simulink model "FOSWEC2"  (R2025b)
settings: Solver=FixedStepAuto  StartTime=0.0  StopTime=Inf  FixedStep=Ts  RelTol=1e-3
values from neighbouring files (symbols this model uses):
  ExcelGains = table2array(ExcelGains)    [initFOSWEC2.m]
  gainTstep = 1.55*20    (= 31)    [initFOSWEC2.m]
  stepTime = 10    [initFOSWEC2.m]
  T = 5    [initFOSWEC2.m]
  Ts = 0.001    [initFOSWEC2.m]
undefined symbols (not defined in the file or in its folder): aft, aftBus_V, aftCurrent_A, aftFlap_deg, aftFlap_Nm, aftPos_rad, aftPower_W, aftRotVel_radpers, aftRotVelFilt_radpers, aftRotVelfromPos_radpers, aftTarget_A, aftTarget_Nm, aftTorque_Nm, bow, bowBus_V, bowCurrent_A, bowFlap_deg, bowFlap_Nm, bowPos_rad, bowPower_W, bowRotVel_radpers, bowRotVelFilt_radpers, bowRotVelfromPos_radpers, bowTarget_A, bowTarget_Nm, bowTorque_Nm, rampTime
libraries: slrealtimeethercatlib x30, simulink x20, slrealtimeloglib x10, dspfdesign x4, cstblocks x2, slrealtimeptplib x1, dspsrcs4 x1
settings Model: Creator=HWRL user  LastModifiedBy=bosmab
settings SolverCC: ConcurrentTasks=on  PositivePriorityOrder=on
settings DataIOCC: ExternalInput=ds  LoadExternalInput=on
settings OptimizationCC: BlockReduction=off  OptimizeBlockIOStorage=off  ReuseModelBlockBuffer=off
settings DebuggingCC: TasksWithSamePriorityMsg=none  ParameterPrecisionLossMsg=none
settings HardwareCC: ProdBitPerLong=64.0  ProdLongLongMode=on  ProdHWDeviceType=Intel->x86-64 (Linux 64)
settings RTWCC: SystemTargetFile=speedgoat.tlc  TemplateMakefile=slrealtime_default_tmf  RTWVerbose=off  Toolchain=Simulink Real-Time Toolchain  BuildConfiguration=Faster Runs  CodeExecutionProfiling=on  TargetLang=C++  GPUComputeCapability=3.5  Description=Speedgoat Real-Time Target Machine
settings SimulinkRealTimeTargetCC: SLRTFileLogMaxRuns=1.0  ExtModeMaxTrigDuration=10.0  ExtModeStaticAllocSize=1000000.0  ExtModeTransport=0.0  MultiwordLength=2048.0  DynamicStringBufferSize=256.0  PreserveMATLABNamespacesInGeneratedCode=on  SubcomponentCodeInterfacePackaging=Reusable function  InstructionSetFMA=off  LogToMDFFile=off

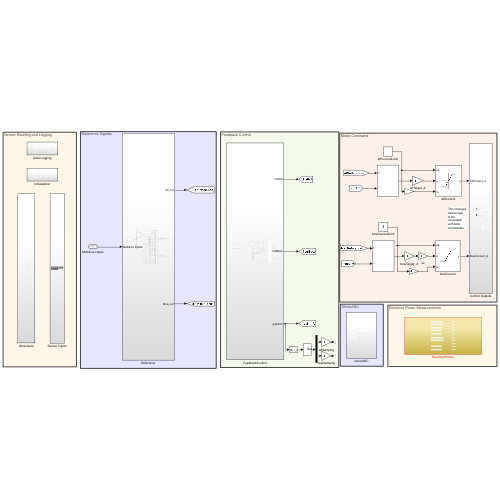
[thumbnail: Simulink's stored preview of the top-level diagram]
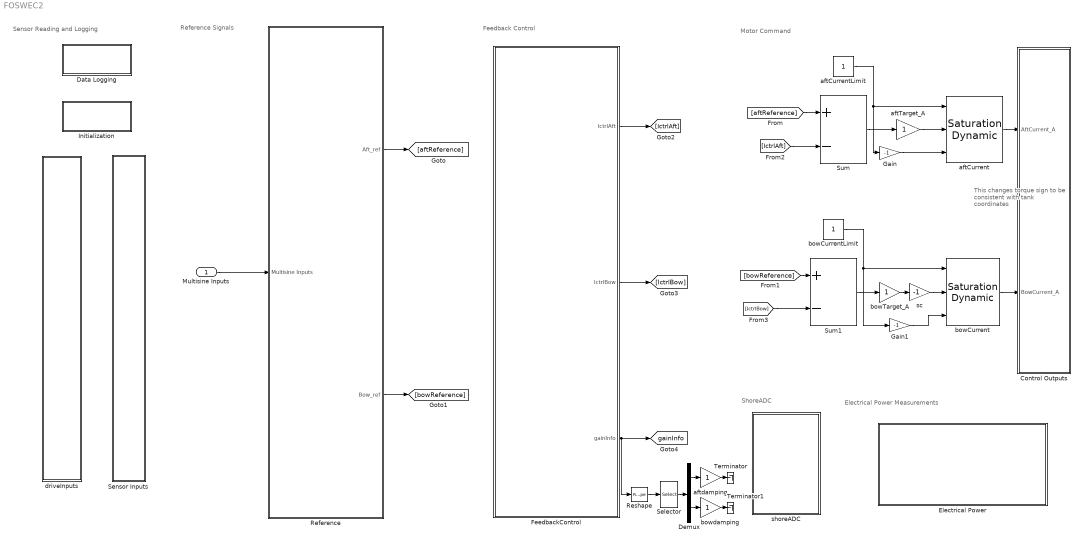
== system FOSWEC2 ==
  note: Electrical Power Measurements
  note: ShoreADC
  note: Sensor Reading and Logging
  note: Motor Command
  note: Feedback Control
  note: Reference Signals
  note: This changes torque sign to be consistent with tank coordinates
  Multisine Inputs : Inport  OutDataTypeStr=Bus: refSigs
  Control Outputs : Subsystem
  Data Logging : Subsystem
  Demux : Demux  Outputs=2
  Electrical Power : Subsystem
  FeedbackControl : Subsystem
  Gain : Gain  Gain=-1
  Gain1 : Gain  Gain=-1
  Initialization : Subsystem
  Reference : Subsystem
  Reshape : Reshape
  Selector : Selector  InputPortWidth=8  IndexOptions=Index vector (dialog)  Indices=[2 8]  OutputSizes=1
  Sensor Inputs : Subsystem
  Sum : Sum  Inputs=+-
  Sum1 : Sum  Inputs=+-
  Terminator : Terminator
  Terminator1 : Terminator
  aftCurrent : simulink/Discontinuities/Saturation Dynamic  OutMin=[]  OutMax=[]  OutDataTypeStr=Inherit: Same as second input  OutDataType=fixdt(1, 16)  OutScaling=2^-10  DoSatur=off
  aftCurrentLimit : Constant
  aftTarget_A : Gain
  aftdamping : Gain
  bowCurrent : simulink/Discontinuities/Saturation Dynamic  OutMin=[]  OutMax=[]  OutDataTypeStr=Inherit: Same as second input  OutDataType=fixdt(1, 16)  OutScaling=2^-10  DoSatur=off
  bowCurrentLimit : Constant
  bowTarget_A : Gain
  bowdamping : Gain
  driveInputs : Subsystem
  sc : Gain  Gain=-1
  shoreADC : Subsystem
  tag scope: gainInfo=global
  wires:
  Sum/1 -> aftTarget_A/1
  Gain/1 -> aftCurrent/3
  aftCurrentLimit/1 -> Gain/1, aftCurrent/1
  [IctrlBow] -> Sum1/2
  bowCurrentLimit/1 -> Gain1/1, bowCurrent/1
  Gain1/1 -> bowCurrent/3
  Sum1/1 -> bowTarget_A/1
  [aftReference] -> Sum/1
  FeedbackControl/1(IctrlAft) -> [IctrlAft]
  [IctrlAft] -> Sum/2
  FeedbackControl/2(IctrlBow) -> [IctrlBow]
  FeedbackControl/3(gainInfo) -> Reshape/1, [gainInfo]
  [bowReference] -> Sum1/1
  bowTarget_A/1 -> sc/1
  aftCurrent/1 -> Control Outputs/1(AftCurrent_A)
  bowCurrent/1 -> Control Outputs/2(BowCurrent_A)
  sc/1 -> bowCurrent/2
  aftTarget_A/1 -> aftCurrent/2
  Demux/1 -> aftdamping/1
  Demux/2 -> bowdamping/1
  aftdamping/1 -> Terminator/1
  bowdamping/1 -> Terminator1/1
  Reshape/1 -> Selector/1
  Selector/1 -> Demux/1
  Multisine Inputs/1 -> Reference/1(Multisine Inputs)
  Reference/1(Aft_ref) -> [aftReference]
  Reference/2(Bow_ref) -> [bowReference]

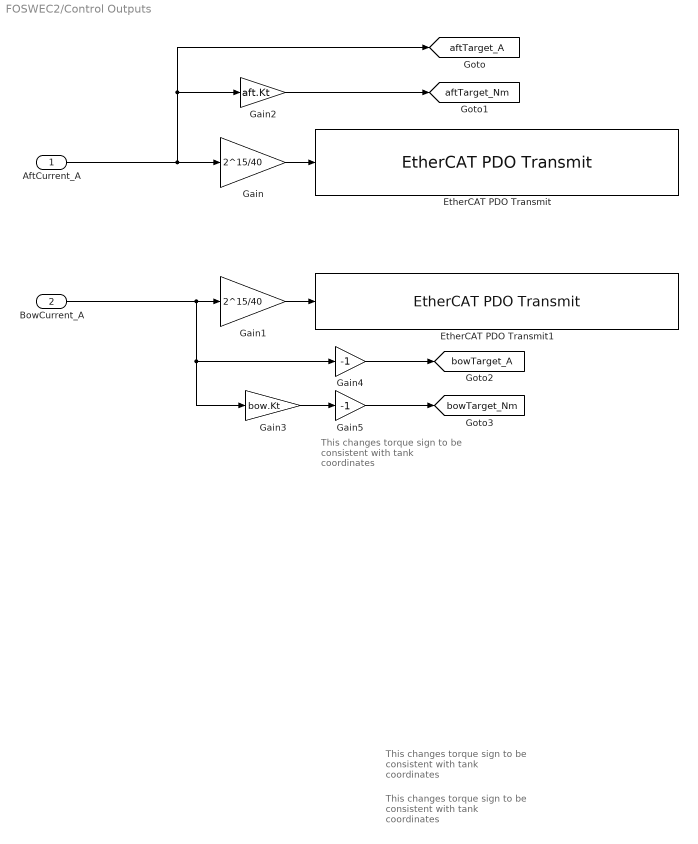
== system FOSWEC2/Control Outputs ==
  note: This changes torque sign to be consistent with tank coordinates
  note: This changes torque sign to be consistent with tank coordinates
  note: This changes torque sign to be consistent with tank coordinates
  AftCurrent_A : Inport
  BowCurrent_A : Inport  Port=2
  EtherCAT PDO Transmit : slrealtimeethercatlib/EtherCAT PDO Transmit  Priority=3  sig_name=Drive 8 (AMC).Module 1 (Default).PDO data to Slave.Target Current  sig_offset=792  sig_type=int16  type_size=16  sig_dim=1  device_id=0  sample_time=0.001000
  EtherCAT PDO Transmit1 : slrealtimeethercatlib/EtherCAT PDO Transmit  Priority=3  sig_name=Drive 4 (AMC).Module 1 (Default).PDO data to Slave.Target Current  sig_offset=648  sig_type=int16  type_size=16  sig_dim=1  device_id=0  sample_time=0.001000
  Gain : Gain  Gain=2^15/40  OutDataTypeStr=int16
  Gain1 : Gain  Gain=2^15/40  OutDataTypeStr=int16
  Gain2 : Gain  Gain=aft.Kt
  Gain3 : Gain  Gain=bow.Kt
  Gain4 : Gain  Gain=-1
  Gain5 : Gain  Gain=-1
  tag scope: aftTarget_A=global, aftTarget_Nm=global, bowTarget_A=global, bowTarget_Nm=global
  wires:
  Gain/1 -> EtherCAT PDO Transmit/1
  Gain1/1 -> EtherCAT PDO Transmit1/1
  Gain2/1 -> [aftTarget_Nm]
  Gain3/1 -> Gain5/1
  BowCurrent_A/1 -> Gain3/1, Gain4/1, Gain1/1
  AftCurrent_A/1 -> Gain/1, [aftTarget_A], Gain2/1
  Gain4/1 -> [bowTarget_A]
  Gain5/1 -> [bowTarget_Nm]

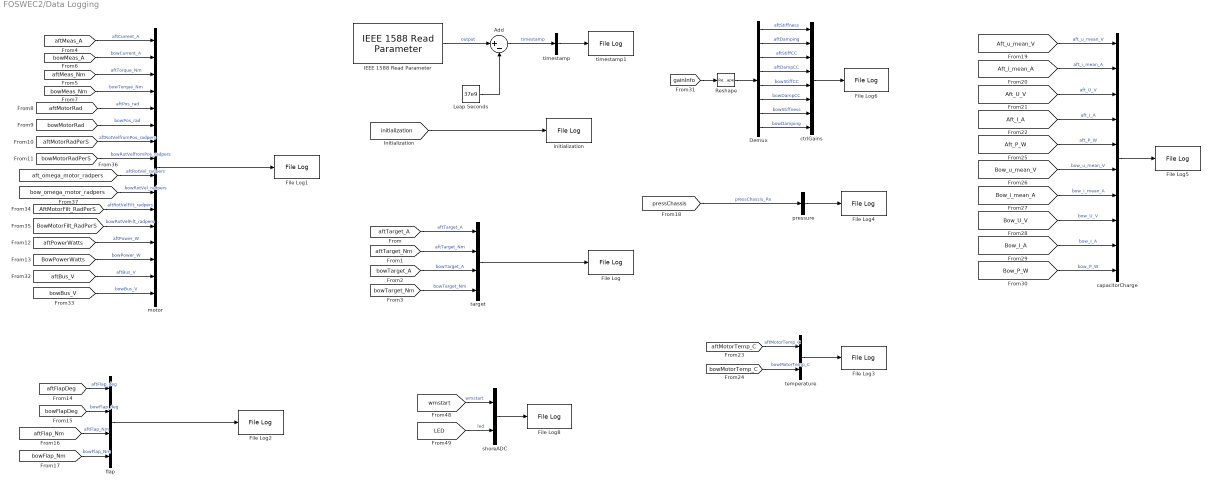
== system FOSWEC2/Data Logging ==
  Add : Sum  Inputs=|+-
  Demux : Demux  Outputs=8
  File Log{,1..6,8} (8 alike) : slrealtimeloglib/File Log  decimation=1  inputProcessing=Elements as channels (sample based)
  IEEE 1588 Read Parameter : slrealtimeptplib/IEEE 1588 Read Parameter  Priority=1  ID=1  param=1. System time (nanosecond)  sample_time=Ts
  Leap Seconds : Constant  Value=37e9
  Reshape : Reshape
  capacitorCharge : BusCreator  Inputs=10
  ctrlGains : BusCreator  Inputs=8
  flap : BusCreator  Inputs=aftFlap_deg,bowFlap_deg,aftFlap_Nm,bowFlap_Nm
  initialization : slrealtimeloglib/File Log  decimation=1  inputProcessing=Elements as channels (sample based)
  motor : BusCreator  Inputs=aftCurrent_A,bowCurrent_A,aftTorque_Nm,bowTorque_Nm,aftPos_rad,bowPos_rad,aftRotVelfromPos_radpers,bowRotVelfromPos_radpers,aftRotVel_radpers,bowRotVel_radpers,aftRotVelFilt_radpers,bowRotVelFilt_radpers,aftPower_W,bowPower_W,aftBus_V,bowBus_V
  pressure : BusCreator  Inputs=1
  shoreADC : BusCreator  Inputs=2
  target : BusCreator  Inputs=aftTarget_A,aftTarget_Nm,bowTarget_A,bowTarget_Nm
  temperature : BusCreator  Inputs=2
  timestamp : BusCreator  Inputs=timestamp
  timestamp1 : slrealtimeloglib/File Log  decimation=1  inputProcessing=Elements as channels (sample based)
  wires:
  Leap Seconds/1 -> Add/2
  IEEE 1588 Read Parameter/1 -> Add/1  "output"
  Add/1 -> timestamp/1  "timestamp"
  timestamp/1 -> timestamp1/1
  [initialization] -> initialization/1
  [aftTarget_A] -> target/1  "aftTarget_A"
  [aftTarget_Nm] -> target/2  "aftTarget_Nm"
  [bowTarget_A] -> target/3  "bowTarget_A"
  [bowTarget_Nm] -> target/4  "bowTarget_Nm"
  target/1 -> File Log/1
  [aftMeas_A] -> motor/1  "aftCurrent_A"
  [aftMeas_Nm] -> motor/3  "aftTorque_Nm"
  [bowMeas_A] -> motor/2  "bowCurrent_A"
  [bowMeas_Nm] -> motor/4  "bowTorque_Nm"
  [aftMotorRad] -> motor/5  "aftPos_rad"
  [bowMotorRad] -> motor/6  "bowPos_rad"
  motor/1 -> File Log1/1
  [aftMotorRadPerS] -> motor/7  "aftRotVelfromPos_radpers"
  [bowMotorRadPerS] -> motor/8  "bowRotVelfromPos_radpers"
  [aftPowerWatts] -> motor/13  "aftPower_W"
  [BowPowerWatts] -> motor/14  "bowPower_W"
  [aftMotorTemp_C] -> temperature/1  "aftMotorTemp_C"
  [bowMotorTemp_C] -> temperature/2  "bowMotorTemp_C"
  temperature/1 -> File Log3/1
  [gainInfo] -> Reshape/1
  Reshape/1 -> Demux/1
  Demux/1 -> ctrlGains/1  "aftStiffness"
  Demux/2 -> ctrlGains/2  "aftDamping"
  Demux/3 -> ctrlGains/3  "aftStiffCC"
  Demux/4 -> ctrlGains/4  "aftDampCC"
  Demux/5 -> ctrlGains/5  "bowStiffCC"
  Demux/6 -> ctrlGains/6  "bowDampCC"
  Demux/7 -> ctrlGains/7  "bowStiffness"
  Demux/8 -> ctrlGains/8  "bowDamping"
  ctrlGains/1 -> File Log6/1
  [aftBus_V] -> motor/15  "aftBus_V"
  [bowBus_V] -> motor/16  "bowBus_V"
  [AftMotorFilt_RadPerS] -> motor/11  "aftRotVelFilt_radpers"
  [BowMotorFilt_RadPerS] -> motor/12  "bowRotVelFilt_radpers"
  [bow_omega_motor_radpers] -> motor/10  "bowRotVel_radpers"
  [aft_omega_motor_radpers] -> motor/9  "aftRotVel_radpers"
  [wmstart] -> shoreADC/1  "wmstart"
  [LED] -> shoreADC/2  "led"
  shoreADC/1 -> File Log8/1
  [aftFlapDeg] -> flap/1  "aftFlap_deg"
  [bowFlapDeg] -> flap/2  "bowFlap_deg"
  flap/1 -> File Log2/1
  [aftFlap_Nm] -> flap/3  "aftFlap_Nm"
  [bowFlap_Nm] -> flap/4  "bowFlap_Nm"
  [pressChassis] -> pressure/1  "pressChassis_Pa"
  pressure/1 -> File Log4/1
  [Aft_u_mean_V] -> capacitorCharge/1  "aft_u_mean_V"
  [Aft_i_mean_A] -> capacitorCharge/2  "aft_i_mean_A"
  [Aft_U_V] -> capacitorCharge/3  "aft_U_V"
  [Aft_I_A] -> capacitorCharge/4  "aft_I_A"
  [Aft_P_W] -> capacitorCharge/5  "aft_P_W"
  [Bow_u_mean_V] -> capacitorCharge/6  "bow_u_mean_V"
  [Bow_i_mean_A] -> capacitorCharge/7  "bow_i_mean_A"
  [Bow_U_V] -> capacitorCharge/8  "bow_U_V"
  [Bow_I_A] -> capacitorCharge/9  "bow_I_A"
  [Bow_P_W] -> capacitorCharge/10  "bow_P_W"
  capacitorCharge/1 -> File Log5/1

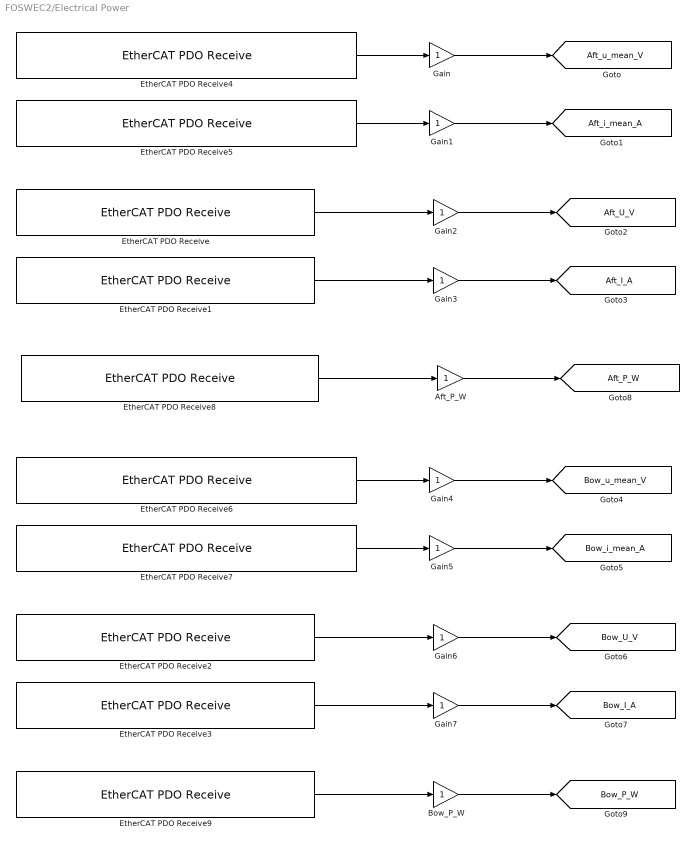
== system FOSWEC2/Electrical Power ==
  Aft_P_W : Gain  OutDataTypeStr=double
  Bow_P_W : Gain  OutDataTypeStr=double
  EtherCAT PDO Receive : slrealtimeethercatlib/EtherCAT PDO Receive  Priority=2  sig_name=Box 1 (GEN Series DAQ System).AftFlap.out.U.AftFlap.out.U_V  sig_offset=2096  sig_type=single  type_size=32  sig_dim=1  device_id=0  sample_time=0.001000
  EtherCAT PDO Receive1 : slrealtimeethercatlib/EtherCAT PDO Receive  Priority=2  sig_name=Box 1 (GEN Series DAQ System).AftFlap.out.I.AftFlap.out.I_V  sig_offset=2056  sig_type=single  type_size=32  sig_dim=1  device_id=0  sample_time=0.001000
  EtherCAT PDO Receive2 : slrealtimeethercatlib/EtherCAT PDO Receive  Priority=2  sig_name=Box 1 (GEN Series DAQ System).BowFlap.out.U.BowFlap.out.U_V  sig_offset=1776  sig_type=single  type_size=32  sig_dim=1  device_id=0  sample_time=0.001
  EtherCAT PDO Receive3 : slrealtimeethercatlib/EtherCAT PDO Receive  Priority=2  sig_name=Box 1 (GEN Series DAQ System).BowFlap.out.I.BowFlap.out.I_V  sig_offset=1736  sig_type=single  type_size=32  sig_dim=1  device_id=0  sample_time=0.001
  EtherCAT PDO Receive4 : slrealtimeethercatlib/EtherCAT PDO Receive  Priority=2  sig_name=Box 1 (GEN Series DAQ System).AftFlap.out.u_mean.AftFlap.out.u_mean_V  sig_offset=2176  sig_type=single  type_size=32  sig_dim=1  device_id=0  sample_time=0.001000
  EtherCAT PDO Receive5 : slrealtimeethercatlib/EtherCAT PDO Receive  Priority=2  sig_name=Box 1 (GEN Series DAQ System).AftFlap.out.i_mean.AftFlap.out.i_mean_V  sig_offset=2136  sig_type=single  type_size=32  sig_dim=1  device_id=0  sample_time=0.001000
  EtherCAT PDO Receive6 : slrealtimeethercatlib/EtherCAT PDO Receive  Priority=2  sig_name=Box 1 (GEN Series DAQ System).BowFlap.out.u_mean.BowFlap.out.u_mean_V  sig_offset=1856  sig_type=single  type_size=32  sig_dim=1  device_id=0  sample_time=0.001
  EtherCAT PDO Receive7 : slrealtimeethercatlib/EtherCAT PDO Receive  Priority=2  sig_name=Box 1 (GEN Series DAQ System).BowFlap.out.i_mean.BowFlap.out.i_mean_V  sig_offset=1816  sig_type=single  type_size=32  sig_dim=1  device_id=0  sample_time=0.001
  EtherCAT PDO Receive8 : slrealtimeethercatlib/EtherCAT PDO Receive  Priority=2  sig_name=Box 1 (GEN Series DAQ System).AftFlap.out.P.AftFlap.out.P_V  sig_offset=2216  sig_type=single  type_size=32  sig_dim=1  device_id=0  sample_time=0.001000
  EtherCAT PDO Receive9 : slrealtimeethercatlib/EtherCAT PDO Receive  Priority=2  sig_name=Box 1 (GEN Series DAQ System).BowFlap.out.P.BowFlap.out.P_V  sig_offset=1896  sig_type=single  type_size=32  sig_dim=1  device_id=0  sample_time=0.001
  Gain{,1..7} (8 alike) : Gain  OutDataTypeStr=double
  tag scope: Aft_I_A=global, Aft_P_W=global, Aft_U_V=global, Aft_i_mean_A=global, Aft_u_mean_V=global, Bow_I_A=global, Bow_P_W=global, Bow_U_V=global, Bow_i_mean_A=global, Bow_u_mean_V=global
  wires:
  Gain/1 -> [Aft_u_mean_V]
  EtherCAT PDO Receive4/1 -> Gain/1
  Gain1/1 -> [Aft_i_mean_A]
  EtherCAT PDO Receive5/1 -> Gain1/1
  EtherCAT PDO Receive1/1 -> Gain3/1
  Gain3/1 -> [Aft_I_A]
  EtherCAT PDO Receive/1 -> Gain2/1
  Gain2/1 -> [Aft_U_V]
  Gain6/1 -> [Bow_U_V]
  EtherCAT PDO Receive2/1 -> Gain6/1
  Gain7/1 -> [Bow_I_A]
  EtherCAT PDO Receive3/1 -> Gain7/1
  EtherCAT PDO Receive7/1 -> Gain5/1
  Gain5/1 -> [Bow_i_mean_A]
  EtherCAT PDO Receive6/1 -> Gain4/1
  Gain4/1 -> [Bow_u_mean_V]
  Aft_P_W/1 -> [Aft_P_W]
  EtherCAT PDO Receive8/1 -> Aft_P_W/1
  EtherCAT PDO Receive9/1 -> Bow_P_W/1
  Bow_P_W/1 -> [Bow_P_W]

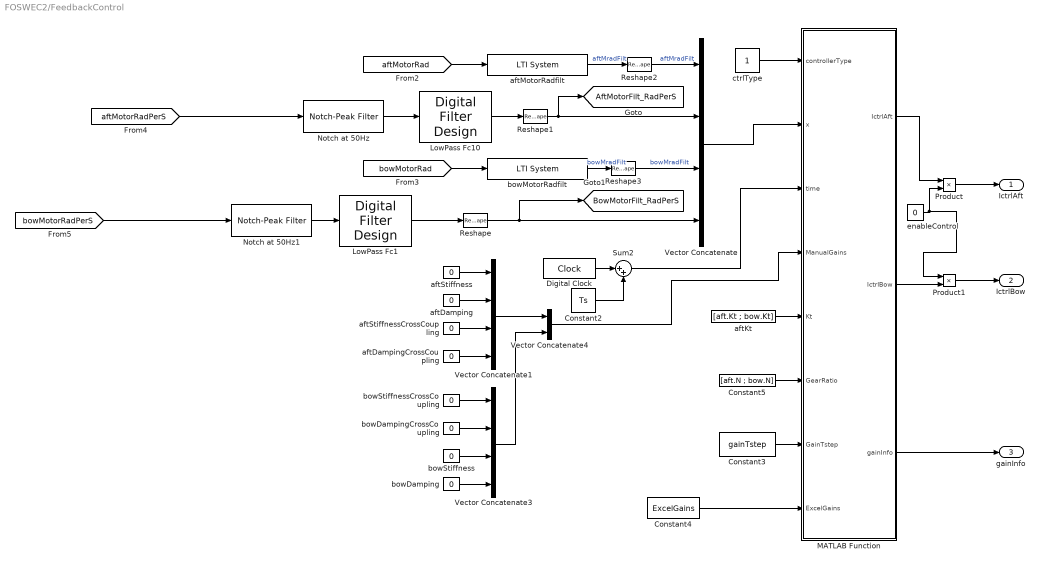
== system FOSWEC2/FeedbackControl ==
  Constant2 : Constant  Value=Ts
  Constant3 : Constant  Value=gainTstep
  Constant4 : Constant  Value=ExcelGains
  Constant5 : Constant  Value=[aft.N ; bow.N]
  Digital Clock : DigitalClock  SampleTime=Ts
  LowPass Fc1 : dspfdesign/Digital Filter Design  mwdsp_browser_bugfix_var=off
  LowPass Fc10 : dspfdesign/Digital Filter Design  mwdsp_browser_bugfix_var=off
  MATLAB Function : MATLAB Function  TreatAsAtomicUnit=on
  Notch at 50Hz : dspfdesign/Notch-Peak Filter  Specification=Bandwidth and center frequency  BandwidthPort=off  Bandwidth=10  QualityFactorPort=off  QualityFactor=5  CenterFrequencyPort=off  CenterFrequency=50  BandwidthCoefficientPort=off  BandwidthCoefficient=0.72654  CenterFrequencyCoefficientPort=off  CenterFrequencyCoefficient=0  Output=Notch  SampleRateMode=Specify on dialog  SampleRate=1000  SimulateUsing=Code generation
  Notch at 50Hz1 : dspfdesign/Notch-Peak Filter  Specification=Bandwidth and center frequency  BandwidthPort=off  Bandwidth=10  QualityFactorPort=off  QualityFactor=5  CenterFrequencyPort=off  CenterFrequency=50  BandwidthCoefficientPort=off  BandwidthCoefficient=0.72654  CenterFrequencyCoefficientPort=off  CenterFrequencyCoefficient=0  Output=Notch  SampleRateMode=Specify on dialog  SampleRate=1000  SimulateUsing=Code generation
  Product : Product
  Product1 : Product
  Reshape{,1..3} (4 alike) : Reshape
  Sum2 : Sum  Inputs=|++
  Vector Concatenate : Concatenate  NumInputs=4  Mode=Multidimensional array
  Vector Concatenate1 : Concatenate  NumInputs=4  Mode=Multidimensional array  ConcatenateDimension=2
  Vector Concatenate3 : Concatenate  NumInputs=4  Mode=Multidimensional array  ConcatenateDimension=2
  Vector Concatenate4 : Concatenate  Mode=Multidimensional array
  aftDamping : Constant  Value=0
  aftDampingCrossCoupling : Constant  Value=0
  aftKt : Constant  Value=[aft.Kt ; bow.Kt]
  aftMotorRadfilt : cstblocks/LTI System  sys=bandpass_dt  IC=[]  PadeOrder=0
  aftStiffness : Constant  Value=0
  aftStiffnessCrossCoupling : Constant  Value=0
  bowDamping : Constant  Value=0
  bowDampingCrossCoupling : Constant  Value=0
  bowMotorRadfilt : cstblocks/LTI System  sys=bandpass_dt  IC=[]  PadeOrder=0
  bowStiffness : Constant  Value=0
  bowStiffnessCrossCoupling : Constant  Value=0
  ctrlType : Constant
  enableControl : Constant  Value=0
  IctrlAft : Outport
  IctrlBow : Outport  Port=2
  gainInfo : Outport  Port=3
  tag scope: AftMotorFilt_RadPerS=global, BowMotorFilt_RadPerS=global
  wires:
  Sum2/1 -> MATLAB Function/3(time)
  Digital Clock/1 -> Sum2/1
  MATLAB Function/1(IctrlAft) -> Product/1
  ctrlType/1 -> MATLAB Function/1(controllerType)
  aftDamping/1 -> Vector Concatenate1/2
  bowStiffness/1 -> Vector Concatenate3/3
  bowDamping/1 -> Vector Concatenate3/4
  bowDampingCrossCoupling/1 -> Vector Concatenate3/2
  Product/1 -> IctrlAft/1
  bowStiffnessCrossCoupling/1 -> Vector Concatenate3/1
  aftDampingCrossCoupling/1 -> Vector Concatenate1/4
  Reshape3/1 -> Vector Concatenate/3  "bowMradFilt"
  Vector Concatenate1/1 -> Vector Concatenate4/1
  [aftMotorRad] -> aftMotorRadfilt/1
  Reshape2/1 -> Vector Concatenate/1  "aftMradFilt"
  MATLAB Function/2(IctrlBow) -> Product1/2
  [bowMotorRad] -> bowMotorRadfilt/1
  aftKt/1 -> MATLAB Function/5(Kt)
  MATLAB Function/3(gainInfo) -> gainInfo/1
  aftStiffness/1 -> Vector Concatenate1/1
  Constant3/1 -> MATLAB Function/7(GainTstep)
  enableControl/1 -> Product1/1, Product/2
  Constant2/1 -> Sum2/2
  aftStiffnessCrossCoupling/1 -> Vector Concatenate1/3
  Vector Concatenate/1 -> MATLAB Function/2(x)
  Constant4/1 -> MATLAB Function/8(ExcelGains)
  Vector Concatenate4/1 -> MATLAB Function/4(ManualGains)
  Vector Concatenate3/1 -> Vector Concatenate4/2
  Constant5/1 -> MATLAB Function/6(GearRatio)
  Product1/1 -> IctrlBow/1
  [aftMotorRadPerS] -> Notch at 50Hz/1
  [bowMotorRadPerS] -> Notch at 50Hz1/1
  Notch at 50Hz/1 -> LowPass Fc10/1
  Notch at 50Hz1/1 -> LowPass Fc1/1
  Reshape1/1 -> [AftMotorFilt_RadPerS], Vector Concatenate/2
  Reshape/1 -> [BowMotorFilt_RadPerS], Vector Concatenate/4
  LowPass Fc1/1 -> Reshape/1
  LowPass Fc10/1 -> Reshape1/1
  aftMotorRadfilt/1 -> Reshape2/1  "aftMradFilt"
  bowMotorRadfilt/1 -> Reshape3/1  "bowMradFilt"

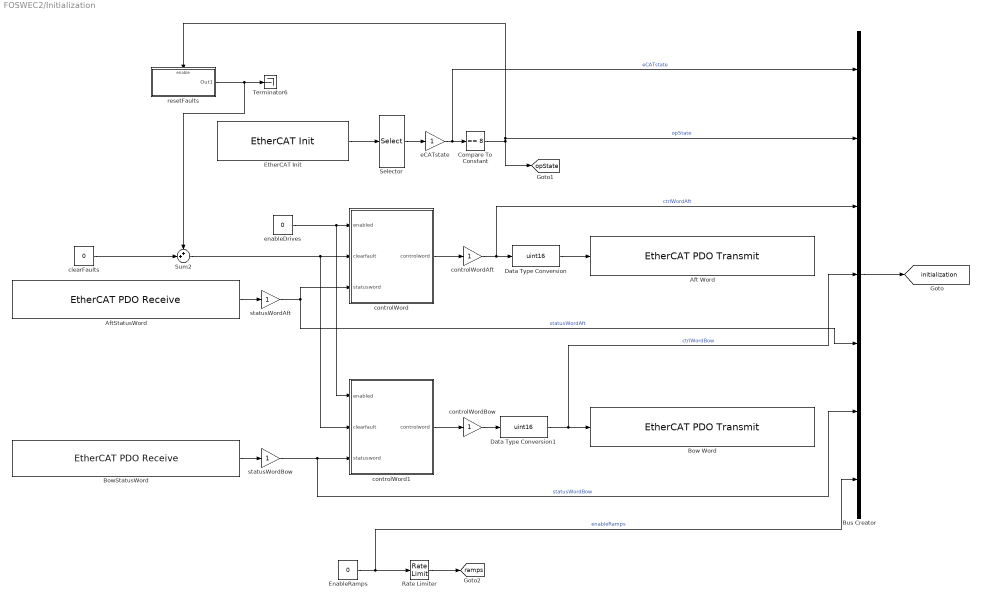
== system FOSWEC2/Initialization ==
  Aft Word : slrealtimeethercatlib/EtherCAT PDO Transmit  Priority=3  sig_name=Drive 8 (AMC).Module 1 (Default).PDO data to Slave.Control Word  sig_offset=712  sig_type=uint16  type_size=16  sig_dim=1  device_id=0  sample_time=0.001000
  AftStatusWord : slrealtimeethercatlib/EtherCAT PDO Receive  Priority=2  sig_name=Drive 8 (AMC).Module 1 (Default).PDO data from Slave.Status Word  sig_offset=712  sig_type=uint16  type_size=16  sig_dim=1  device_id=0  sample_time=0.001000
  Bow Word : slrealtimeethercatlib/EtherCAT PDO Transmit  Priority=3  sig_name=Drive 4 (AMC).Module 1 (Default).PDO data to Slave.Control Word  sig_offset=568  sig_type=uint16  type_size=16  sig_dim=1  device_id=0  sample_time=0.001000
  BowStatusWord : slrealtimeethercatlib/EtherCAT PDO Receive  Priority=2  sig_name=Drive 4 (AMC).Module 1 (Default).PDO data from Slave.Status Word  sig_offset=568  sig_type=uint16  type_size=16  sig_dim=1  device_id=0  sample_time=0.001000
  Bus Creator : BusCreator  Inputs=7
  Compare To Constant : simulink/Logic and Bit Operations/Compare To Constant  relop===  const=8  OutDataTypeStr=boolean
  Data Type Conversion : DataTypeConversion  OutDataTypeStr=uint16  SaturateOnIntegerOverflow=off  RndMeth=Floor
  Data Type Conversion1 : DataTypeConversion  OutDataTypeStr=uint16  SaturateOnIntegerOverflow=off  RndMeth=Floor
  EnableRamps : Constant  Value=0  OutDataTypeStr=Inherit: Inherit via back propagation
  EtherCAT Init : slrealtimeethercatlib/EtherCAT Init  Priority=0  config_file=C:\Software\FOSWEC2\Simulink\..\TwinCAT\NAVFACOSWECSxml.xml  device_id=0  portnum=1  initstate=2  dctuning=0  enaDebug=0  logFile='c:\dbglog.txt'  sample_time=0.001000  DCMode=2
  Rate Limiter : RateLimiter  RisingSlewLimit=1/rampTime  FallingSlewLimit=-1/rampTime  SampleTimeMode=inherited
  Selector : Selector  InputPortWidth=6  IndexOptions=Index vector (dialog)  Indices=[2]  OutputSizes=1
  Sum2 : Sum  Inputs=++|
  Terminator6 : Terminator
  clearFaults : Constant  Value=0
  controlWord : MATLAB Function  TreatAsAtomicUnit=on
  controlWord1 : MATLAB Function  TreatAsAtomicUnit=on
  controlWordAft : Gain  OutDataTypeStr=double
  controlWordBow : Gain  OutDataTypeStr=double
  eCATstate : Gain  OutDataTypeStr=double
  enableDrives : Constant  Value=0
  resetFaults : Subsystem  TreatAsAtomicUnit=on
  statusWordAft : Gain  OutDataTypeStr=double
  statusWordBow : Gain  OutDataTypeStr=double
  tag scope: initialization=global, opState=global, ramps=global
  wires:
  EtherCAT Init/1 -> Selector/1
  Selector/1 -> eCATstate/1
  eCATstate/1 -> Bus Creator/1, Compare To Constant/1  "eCATstate"
  Compare To Constant/1 -> resetFaults/Enable, Bus Creator/2, [opState]  "opState"
  Bus Creator/1 -> [initialization]
  AftStatusWord/1 -> statusWordAft/1
  BowStatusWord/1 -> statusWordBow/1
  statusWordBow/1 -> Bus Creator/6, controlWord1/3(statusword)  "statusWordBow"
  statusWordAft/1 -> controlWord/3(statusword), Bus Creator/5  "statusWordAft"
  Data Type Conversion/1 -> Aft Word/1
  enableDrives/1 -> controlWord1/1(enabled), controlWord/1(enabled)
  Sum2/1 -> controlWord1/2(clearfault), controlWord/2(clearfault)
  controlWord/1(controlword) -> controlWordAft/1
  controlWordAft/1 -> Bus Creator/3, Data Type Conversion/1  "ctrlWordAft"
  controlWord1/1(controlword) -> controlWordBow/1
  controlWordBow/1 -> Data Type Conversion1/1
  Data Type Conversion1/1 -> Bus Creator/4, Bow Word/1  "ctrlWordBow"
  resetFaults/1(Out1) -> Terminator6/1, Sum2/1
  clearFaults/1 -> Sum2/2
  EnableRamps/1 -> Bus Creator/7, Rate Limiter/1  "enableRamps"
  Rate Limiter/1 -> [ramps]

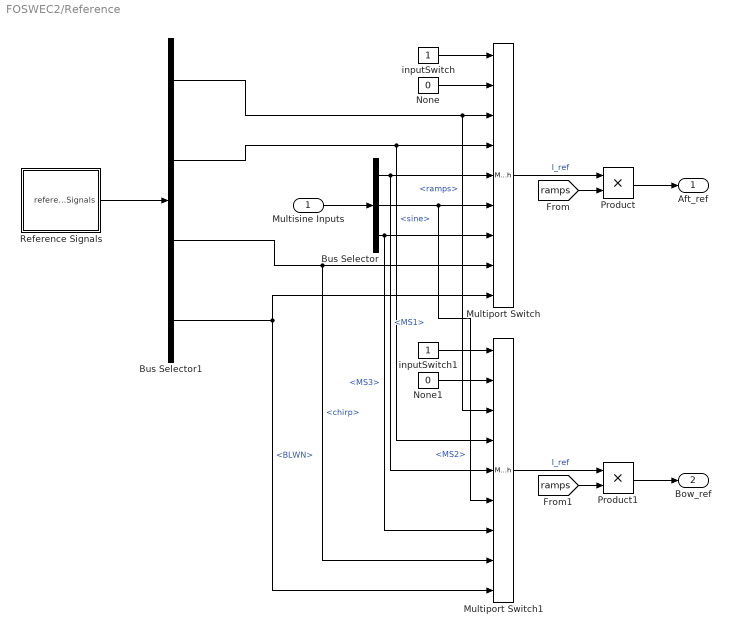
== system FOSWEC2/Reference ==
  Multisine Inputs : Inport
  Bus Selector : BusSelector  OutputSignals=MS1,MS2,MS3
  Bus Selector1 : BusSelector  OutputSignals=ramps,sine,chirp,BLWN
  Multiport Switch : MultiPortSwitch  Inputs=8  SaturateOnIntegerOverflow=off  InputSameDT=off
  Multiport Switch1 : MultiPortSwitch  Inputs=8  SaturateOnIntegerOverflow=off  InputSameDT=off
  None : Constant  Value=0
  None1 : Constant  Value=0
  Product : Product
  Product1 : Product
  Reference Signals : Subsystem
  inputSwitch : Constant
  inputSwitch1 : Constant
  Aft_ref : Outport
  Bow_ref : Outport  Port=2
  wires:
  inputSwitch/1 -> Multiport Switch/1
  Bus Selector/3 -> Multiport Switch/7, Multiport Switch1/7  "<MS3>"
  Reference Signals/1(referenceSignals) -> Bus Selector1/1
  Bus Selector/2 -> Multiport Switch1/6, Multiport Switch/6  "<MS2>"
  Bus Selector1/2 -> Multiport Switch/4, Multiport Switch1/4  "<sine>"
  Bus Selector1/4 -> Multiport Switch1/9, Multiport Switch/9  "<BLWN>"
  Bus Selector1/3 -> Multiport Switch1/8, Multiport Switch/8  "<chirp>"
  None/1 -> Multiport Switch/2
  Bus Selector/1 -> Multiport Switch/5, Multiport Switch1/5  "<MS1>"
  Bus Selector1/1 -> Multiport Switch1/3, Multiport Switch/3  "<ramps>"
  Multiport Switch/1 -> Product/1  "I_ref"
  Multisine Inputs/1 -> Bus Selector/1
  None1/1 -> Multiport Switch1/2
  inputSwitch1/1 -> Multiport Switch1/1
  Product/1 -> Aft_ref/1
  [ramps] -> Product/2
  [ramps] -> Product1/2
  Multiport Switch1/1 -> Product1/1  "I_ref"
  Product1/1 -> Bow_ref/1

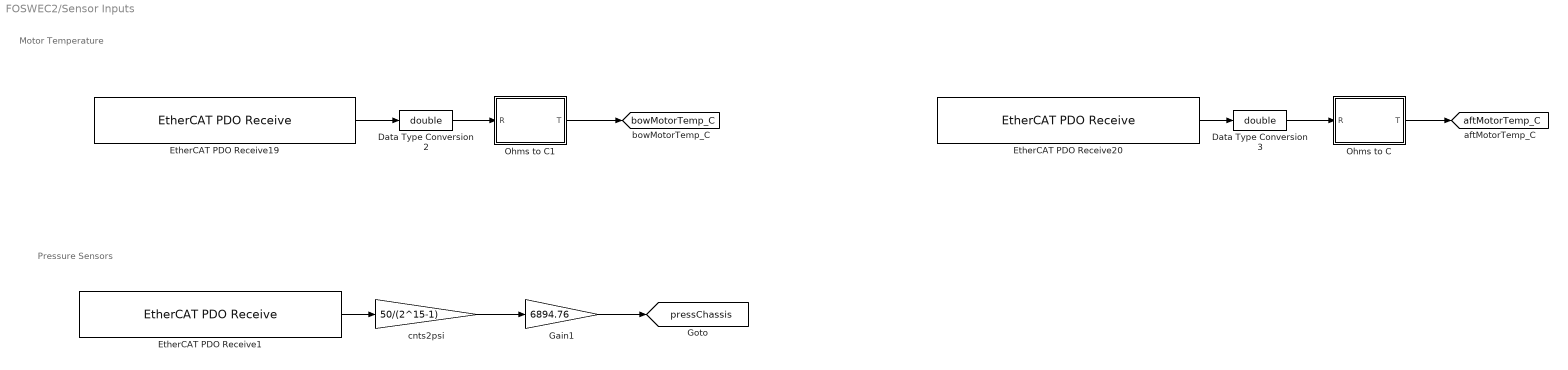
== system FOSWEC2/Sensor Inputs ==
  note: Pressure Sensors
  note: Motor Temperature
  Data Type Conversion2 : DataTypeConversion  OutDataTypeStr=double  SaturateOnIntegerOverflow=off  RndMeth=Floor
  Data Type Conversion3 : DataTypeConversion  OutDataTypeStr=double  SaturateOnIntegerOverflow=off  RndMeth=Floor
  EtherCAT PDO Receive1 : slrealtimeethercatlib/EtherCAT PDO Receive  Priority=2  sig_name=Term 6 (EL3154).AI Standard Channel 1.Value  sig_offset=1096  sig_type=int16  type_size=16  sig_dim=1  device_id=0  sample_time=0.001000
  EtherCAT PDO Receive19 : slrealtimeethercatlib/EtherCAT PDO Receive  Priority=2  sig_name=Term 7 (EL3692).SAI Inputs Channel 1.Value  sig_offset=1224  sig_type=int32  type_size=32  sig_dim=1  device_id=0  sample_time=0.001000
  EtherCAT PDO Receive20 : slrealtimeethercatlib/EtherCAT PDO Receive  Priority=2  sig_name=Term 7 (EL3692).SAI Inputs Channel 2.Value  sig_offset=1320  sig_type=int32  type_size=32  sig_dim=1  device_id=0  sample_time=0.001000
  Gain1 : Gain  Gain=6894.76
  Ohms to C : MATLAB Function  TreatAsAtomicUnit=on
  Ohms to C1 : MATLAB Function  TreatAsAtomicUnit=on
  cnts2psi : Gain  Gain=50/(2^15-1)  OutDataTypeStr=double
  tag scope: aftMotorTemp_C=global, bowMotorTemp_C=global, pressChassis=global
  wires:
  EtherCAT PDO Receive19/1 -> Data Type Conversion2/1
  EtherCAT PDO Receive20/1 -> Data Type Conversion3/1
  Data Type Conversion3/1 -> Ohms to C/1(R)
  Ohms to C/1(T) -> [aftMotorTemp_C]
  Data Type Conversion2/1 -> Ohms to C1/1(R)
  Ohms to C1/1(T) -> [bowMotorTemp_C]
  EtherCAT PDO Receive1/1 -> cnts2psi/1
  cnts2psi/1 -> Gain1/1
  Gain1/1 -> [pressChassis]

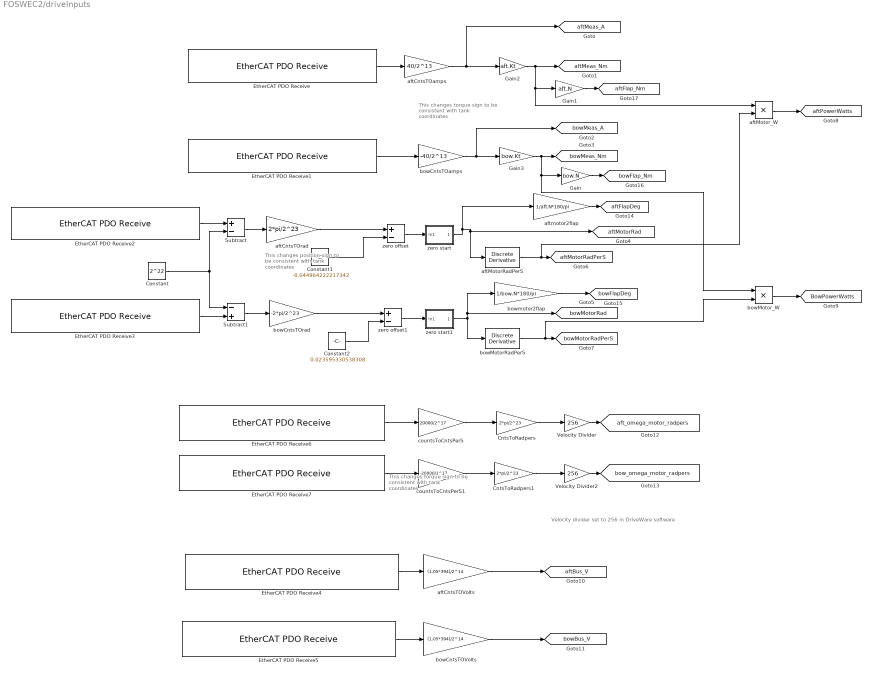
== system FOSWEC2/driveInputs ==
  note: Velocity divider set to 256 in DriveWare software
  note: This changes torque sign to be consistent with tank coordinates
  note: This changes position sign to be consistent with tank coordinates
  note: This changes torque sign to be consistent with tank coordinates
  CntsToRadpers : Gain  Gain=2*pi/2^23
  CntsToRadpers1 : Gain  Gain=2*pi/2^23
  Constant : Constant  Value=2^22
  Constant1 : Constant  Value=-0.044964222217342
  Constant2 : Constant  Value=0.023595330538308
  EtherCAT PDO Receive : slrealtimeethercatlib/EtherCAT PDO Receive  Priority=2  sig_name=Drive 8 (AMC).Module 1 (Default).PDO data from Slave.Actual Current  sig_offset=792  sig_type=int16  type_size=16  sig_dim=1  device_id=0  sample_time=0.001000
  EtherCAT PDO Receive1 : slrealtimeethercatlib/EtherCAT PDO Receive  Priority=2  sig_name=Drive 4 (AMC).Module 1 (Default).PDO data from Slave.Actual Current  sig_offset=648  sig_type=int16  type_size=16  sig_dim=1  device_id=0  sample_time=0.001000
  EtherCAT PDO Receive2 : slrealtimeethercatlib/EtherCAT PDO Receive  Priority=2  sig_name=Drive 8 (AMC).Module 1 (Default).PDO data from Slave.Actual position  sig_offset=728  sig_type=int32  type_size=32  sig_dim=1  device_id=0  sample_time=0.001000
  EtherCAT PDO Receive3 : slrealtimeethercatlib/EtherCAT PDO Receive  Priority=2  sig_name=Drive 4 (AMC).Module 1 (Default).PDO data from Slave.Actual position  sig_offset=584  sig_type=int32  type_size=32  sig_dim=1  device_id=0  sample_time=0.001000
  EtherCAT PDO Receive4 : slrealtimeethercatlib/EtherCAT PDO Receive  Priority=2  sig_name=Drive 8 (AMC).Module 1 (Default).PDO data from Slave.DC Bus Voltage  sig_offset=824  sig_type=uint16  type_size=16  sig_dim=1  device_id=0  sample_time=0.001000
  EtherCAT PDO Receive5 : slrealtimeethercatlib/EtherCAT PDO Receive  Priority=2  sig_name=Drive 4 (AMC).Module 1 (Default).PDO data from Slave.DC Bus Voltage  sig_offset=680  sig_type=uint16  type_size=16  sig_dim=1  device_id=0  sample_time=0.001000
  EtherCAT PDO Receive6 : slrealtimeethercatlib/EtherCAT PDO Receive  Priority=2  sig_name=Drive 8 (AMC).Module 1 (Default).PDO data from Slave.Actual Velocity  sig_offset=760  sig_type=int32  type_size=32  sig_dim=1  device_id=0  sample_time=0.001000
  EtherCAT PDO Receive7 : slrealtimeethercatlib/EtherCAT PDO Receive  Priority=2  sig_name=Drive 4 (AMC).Module 1 (Default).PDO data from Slave.Actual Velocity  sig_offset=616  sig_type=int32  type_size=32  sig_dim=1  device_id=0  sample_time=0.001000
  Gain : Gain  Gain=bow.N
  Gain1 : Gain  Gain=aft.N
  Gain2 : Gain  Gain=aft.Kt  ParamDataTypeStr=double  OutDataTypeStr=double
  Gain3 : Gain  Gain=bow.Kt  ParamDataTypeStr=double  OutDataTypeStr=double
  Subtract : Sum  Inputs=+-
  Subtract1 : Sum  Inputs=-+
  Velocity Divider : Gain  Gain=256
  Velocity Divider2 : Gain  Gain=256
  aftCntsTOVolts : Gain  Gain=(1.05*394)/2^14  OutDataTypeStr=double
  aftCntsTOamps : Gain  Gain=40/2^13  OutDataTypeStr=double
  aftCntsTOrad : Gain  Gain=2*pi/2^23  ParamDataTypeStr=double  OutDataTypeStr=double
  aftMotorRadPerS : simulink/Discrete/Discrete Derivative  gainval=1.0  ICPrevScaledInput=0.0  OutMin=[]  OutMax=[]  OutDataType=fixdt(1, 16)  OutScaling=2^-10  DoSatur=off
  aftMotor_W : Product
  aftmotor2flap : Gain  Gain=1/aft.N*180/pi
  bowCntsTOVolts : Gain  Gain=(1.05*394)/2^14  OutDataTypeStr=double
  bowCntsTOamps : Gain  Gain=-40/2^13  OutDataTypeStr=double
  bowCntsTOrad : Gain  Gain=-2*pi/2^23  ParamDataTypeStr=double  OutDataTypeStr=double
  bowMotorRadPerS : simulink/Discrete/Discrete Derivative  gainval=1.0  ICPrevScaledInput=0.0  OutMin=[]  OutMax=[]  OutDataType=fixdt(1, 16)  OutScaling=2^-10  DoSatur=off
  bowMotor_W : Product
  bowmotor2flap : Gain  Gain=1/bow.N*180/pi
  countsToCntsPerS : Gain  Gain=20000/2^17  OutDataTypeStr=double
  countsToCntsPerS1 : Gain  Gain=-20000/2^17  OutDataTypeStr=double
  zero offset : Sum  Inputs=+-
  zero offset1 : Sum  Inputs=+-
  zero start : Subsystem
  zero start1 : Subsystem
  tag scope: BowPowerWatts=global, aftBus_V=global, aftFlapDeg=global, aftFlap_Nm=global, aftMeas_A=global, aftMeas_Nm=global, aftMotorRad=global, aftMotorRadPerS=global, aftPowerWatts=global, aft_omega_motor_radpers=global, bowBus_V=global, bowFlapDeg=global, bowFlap_Nm=global, bowMeas_A=global, bowMeas_Nm=global, bowMotorRad=global, bowMotorRadPerS=global, bow_omega_motor_radpers=global
  wires:
  EtherCAT PDO Receive1/1 -> bowCntsTOamps/1
  EtherCAT PDO Receive/1 -> aftCntsTOamps/1
  bowCntsTOamps/1 -> [bowMeas_A], Gain3/1
  Gain3/1 -> bowMotor_W/1, Gain/1, [bowMeas_Nm]
  aftCntsTOamps/1 -> [aftMeas_A], Gain2/1
  zero offset1/1 -> zero start1/1(In1)
  aftMotorRadPerS/1 -> aftMotor_W/2, [aftMotorRadPerS]
  bowMotorRadPerS/1 -> bowMotor_W/2, [bowMotorRadPerS]
  aftMotor_W/1 -> [aftPowerWatts]
  bowMotor_W/1 -> [BowPowerWatts]
  zero offset/1 -> zero start/1(In1)
  aftmotor2flap/1 -> [aftFlapDeg]
  bowmotor2flap/1 -> [bowFlapDeg]
  EtherCAT PDO Receive4/1 -> aftCntsTOVolts/1
  aftCntsTOVolts/1 -> [aftBus_V]
  EtherCAT PDO Receive5/1 -> bowCntsTOVolts/1
  bowCntsTOVolts/1 -> [bowBus_V]
  EtherCAT PDO Receive6/1 -> countsToCntsPerS/1
  EtherCAT PDO Receive7/1 -> countsToCntsPerS1/1
  countsToCntsPerS/1 -> CntsToRadpers/1
  countsToCntsPerS1/1 -> CntsToRadpers1/1
  CntsToRadpers/1 -> Velocity Divider/1
  CntsToRadpers1/1 -> Velocity Divider2/1
  Velocity Divider/1 -> [aft_omega_motor_radpers]
  Velocity Divider2/1 -> [bow_omega_motor_radpers]
  Gain/1 -> [bowFlap_Nm]
  Gain1/1 -> [aftFlap_Nm]
  Gain2/1 -> Gain1/1, aftMotor_W/1, [aftMeas_Nm]
  EtherCAT PDO Receive2/1 -> Subtract/1
  Constant/1 -> Subtract1/1, Subtract/2
  EtherCAT PDO Receive3/1 -> Subtract1/2
  Subtract/1 -> aftCntsTOrad/1
  Subtract1/1 -> bowCntsTOrad/1
  aftCntsTOrad/1 -> zero offset/1
  Constant1/1 -> zero offset/2
  Constant2/1 -> zero offset1/2
  bowCntsTOrad/1 -> zero offset1/1
  zero start/1(Out1) -> aftmotor2flap/1, aftMotorRadPerS/1, [aftMotorRad]
  zero start1/1(Out1) -> bowmotor2flap/1, [bowMotorRad], bowMotorRadPerS/1

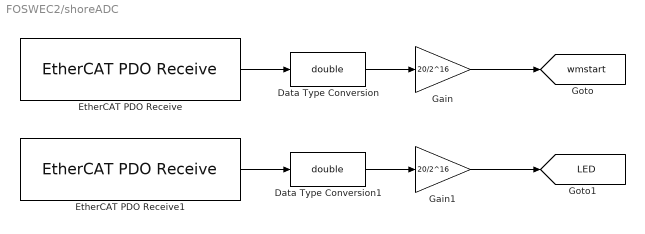
== system FOSWEC2/shoreADC ==
  Data Type Conversion : DataTypeConversion  OutDataTypeStr=double  SaturateOnIntegerOverflow=off  RndMeth=Floor
  Data Type Conversion1 : DataTypeConversion  OutDataTypeStr=double  SaturateOnIntegerOverflow=off  RndMeth=Floor
  EtherCAT PDO Receive : slrealtimeethercatlib/EtherCAT PDO Receive  Priority=2  sig_name=Term 3 (EL3104).AI Standard Channel 1.Value  sig_offset=968  sig_type=int16  type_size=16  sig_dim=1  device_id=0  sample_time=0.001000
  EtherCAT PDO Receive1 : slrealtimeethercatlib/EtherCAT PDO Receive  Priority=2  sig_name=Term 3 (EL3104).AI Standard Channel 2.Value  sig_offset=1000  sig_type=int16  type_size=16  sig_dim=1  device_id=0  sample_time=0.001000
  Gain : Gain  Gain=20/2^16
  Gain1 : Gain  Gain=20/2^16
  tag scope: LED=global, wmstart=global
  wires:
  EtherCAT PDO Receive/1 -> Data Type Conversion/1
  EtherCAT PDO Receive1/1 -> Data Type Conversion1/1
  Data Type Conversion/1 -> Gain/1
  Data Type Conversion1/1 -> Gain1/1
  Gain/1 -> [wmstart]
  Gain1/1 -> [LED]

== system FOSWEC2/Initialization/resetFaults ==
  Enable : EnablePort
  Constant : Constant
  Constant1 : Constant  Value=-1
  Delay : Delay  DelayLength=1000
  Sum : Sum  Inputs=|++
  Out1 : Outport
  wires:
  Constant/1 -> Sum/1
  Constant1/1 -> Delay/1
  Delay/1 -> Sum/2
  Sum/1 -> Out1/1

== system FOSWEC2/Reference/Reference Signals ==
  BLWN : Subsystem
  Bus Creator : BusCreator  Inputs=4
  chirpWave : Subsystem
  ramp : Subsystem
  sineWave : Subsystem
  referenceSignals : Outport
  wires:
  sineWave/1(sineWave) -> Bus Creator/2  "sine"
  BLWN/1(Out1) -> Bus Creator/4  "BLWN"
  chirpWave/1(chirp) -> Bus Creator/3  "chirp"
  Bus Creator/1 -> referenceSignals/1
  ramp/1(ramps) -> Bus Creator/1  "ramps"

== system FOSWEC2/driveInputs/zero start ==
  In1 : Inport
  Switch : Switch  Criteria=u2 > Threshold  SaturateOnIntegerOverflow=off  InputSameDT=off
  Zero : Constant  Value=0  OutDataTypeStr=Inherit: Inherit via back propagation
  Out1 : Outport
  wires:
  Switch/1 -> Out1/1
  In1/1 -> Switch/1
  [opState] -> Switch/2
  Zero/1 -> Switch/3

== system FOSWEC2/driveInputs/zero start1 ==
  In1 : Inport
  Switch : Switch  Criteria=u2 > Threshold  SaturateOnIntegerOverflow=off  InputSameDT=off
  Zero : Constant  Value=0  OutDataTypeStr=Inherit: Inherit via back propagation
  Out1 : Outport
  wires:
  Zero/1 -> Switch/3
  [opState] -> Switch/2
  In1/1 -> Switch/1
  Switch/1 -> Out1/1

== system FOSWEC2/Reference/Reference Signals/BLWN ==
  Band-Limited White Noise : simulink/Sources/Band-Limited White Noise  Cov=[0.0001]  Ts=Ts  seed=[23341]
  Product : Product
  Ramp : simulink/Sources/Ramp  slope=1/(5*T)  start=stepTime  InitialOutput=0
  Ramp1 : simulink/Sources/Ramp  slope=1/(5*T)  start=stepTime+5*T  InitialOutput=0
  Subtract : Sum  Inputs=-+
  Out1 : Outport  OutDataTypeStr=double  PortDimensions=1  SampleTime=0
  wires:
  Ramp1/1 -> Subtract/2
  Subtract/1 -> Product/2
  Ramp/1 -> Subtract/1
  Product/1 -> Out1/1
  Band-Limited White Noise/1 -> Product/1

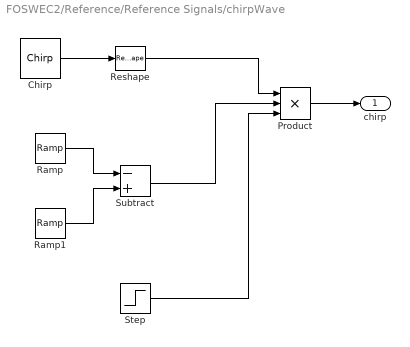
== system FOSWEC2/Reference/Reference Signals/chirpWave ==
  Chirp : dspsrcs4/Chirp  sweep=Linear  mode=Unidirectional  f0=.1  f1=1  t1=300  Tsweep=300  phase=0  Ts=1/1000  spf=1  datatype=double  OutputFrames=off
  Product : Product  Inputs=3
  Ramp : simulink/Sources/Ramp  slope=1/(5*T)  start=2*stepTime  InitialOutput=0
  Ramp1 : simulink/Sources/Ramp  slope=1/(5*T)  start=2*stepTime+5*T  InitialOutput=0
  Reshape : Reshape
  Step : Step  Time=stepTime  SampleTime=0
  Subtract : Sum  Inputs=-+
  chirp : Outport
  wires:
  Ramp1/1 -> Subtract/2
  Ramp/1 -> Subtract/1
  Chirp/1 -> Reshape/1
  Subtract/1 -> Product/2
  Step/1 -> Product/3
  Reshape/1 -> Product/1
  Product/1 -> chirp/1

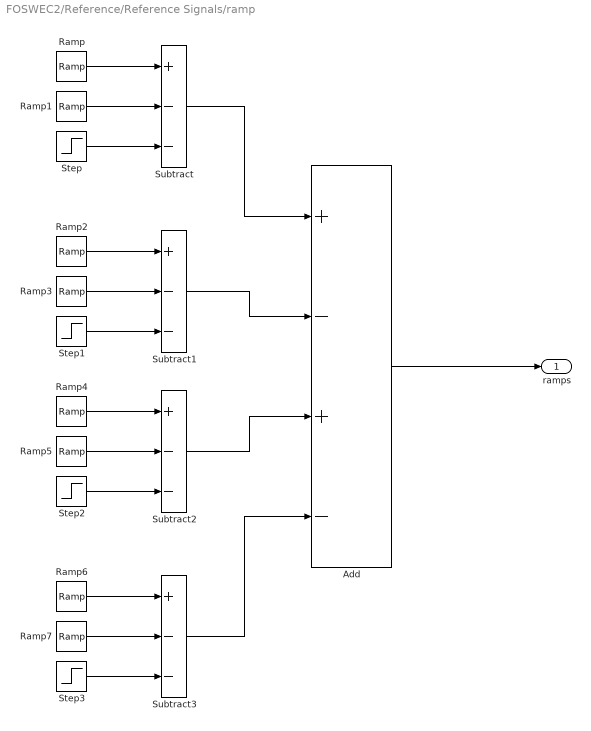
== system FOSWEC2/Reference/Reference Signals/ramp ==
  Add : Sum  Inputs=+-+-
  Ramp : simulink/Sources/Ramp  slope=1/(t(2)-t(1))  start=t(1)  InitialOutput=0
  Ramp1 : simulink/Sources/Ramp  slope=1/(t(2)-t(1))  start=t(2)  InitialOutput=0
  Ramp2 : simulink/Sources/Ramp  slope=1/(t(4)-t(3))  start=t(3)  InitialOutput=0
  Ramp3 : simulink/Sources/Ramp  slope=1/(t(4)-t(3))  start=t(4)  InitialOutput=0
  Ramp4 : simulink/Sources/Ramp  slope=1/(t(6)-t(5))  start=t(5)  InitialOutput=0
  Ramp5 : simulink/Sources/Ramp  slope=1/(t(6)-t(5))  start=t(6)  InitialOutput=0
  Ramp6 : simulink/Sources/Ramp  slope=1/(t(8)-t(7))  start=t(7)  InitialOutput=0
  Ramp7 : simulink/Sources/Ramp  slope=1/(t(8)-t(7))  start=t(8)  InitialOutput=0
  Step : Step  Time=t(2)  SampleTime=0
  Step1 : Step  Time=t(4)  SampleTime=0
  Step2 : Step  Time=t(6)  SampleTime=0
  Step3 : Step  Time=t(8)  SampleTime=0
  Subtract{,1..3} (4 alike) : Sum  Inputs=+--
  ramps : Outport  OutDataTypeStr=double  PortDimensions=1  SampleTime=0
  wires:
  Add/1 -> ramps/1
  Subtract1/1 -> Add/2
  Ramp5/1 -> Subtract2/2
  Ramp/1 -> Subtract/1
  Step1/1 -> Subtract1/3
  Subtract3/1 -> Add/4
  Ramp3/1 -> Subtract1/2
  Ramp2/1 -> Subtract1/1
  Ramp6/1 -> Subtract3/1
  Subtract/1 -> Add/1
  Subtract2/1 -> Add/3
  Step/1 -> Subtract/3
  Step2/1 -> Subtract2/3
  Ramp4/1 -> Subtract2/1
  Ramp1/1 -> Subtract/2
  Step3/1 -> Subtract3/3
  Ramp7/1 -> Subtract3/2

== system FOSWEC2/Reference/Reference Signals/sineWave ==
  Product : Product
  Ramp : simulink/Sources/Ramp  slope=1/(5*T)  start=stepTime  InitialOutput=0
  Ramp1 : simulink/Sources/Ramp  slope=1/(5*T)  start=stepTime+5*T  InitialOutput=0
  Sine Wave : Sin  Frequency=pi  SampleTime=0
  Subtract : Sum  Inputs=-+
  sineWave : Outport  OutDataTypeStr=double  PortDimensions=1  SampleTime=0
  wires:
  Product/1 -> sineWave/1
  Ramp/1 -> Subtract/1
  Sine Wave/1 -> Product/1
  Subtract/1 -> Product/2
  Ramp1/1 -> Subtract/2

== matlab function FOSWEC2/Initialization/controlWord1 ==
  data: enabled input; controlword output; clearfault input; statusword input
function controlword = fcn(enabled, clearfault, statusword)

bitstatus = bitget(statusword,1:16);

if ~clearfault
    if enabled
        if bitstatus(1) == 0 % Ready to switch on not ready
            controlword = 6; % command ready switch on
        elseif ~bitstatus(2) % switched not yet on
            controlword = 7; % command switch on
        elseif ~bitstatus(3) % operation not yet enabled
            controlword = 15; % command enable
        else
            controlword = 15; % maintain enabled state
        end
    else
        controlword = 4; % command disabled
    end
else
    controlword = 128; % command clear faults
end

== matlab function FOSWEC2/Initialization/controlWord ==
  data: enabled input; controlword output; clearfault input; statusword input
function controlword = fcn(enabled, clearfault, statusword)

bitstatus = bitget(statusword,1:16);

if ~clearfault
    if enabled
        if bitstatus(1) == 0 % Ready to switch on not ready
            controlword = 6; % command ready switch on
        elseif ~bitstatus(2) % switched not yet on
            controlword = 7; % command switch on
        elseif ~bitstatus(3) % operation not yet enabled
            controlword = 15; % command enable
        else
            controlword = 15; % maintain enabled state
        end
    else
        controlword = 4; % command disabled
    end
else
    controlword = 128; % command clear faults
end

== matlab function FOSWEC2/Sensor Inputs/Ohms to C ==
  data: R input; T output
function T = ohms2C(R)

R0 = 50000;
B = 3970;
T00 = 273.15;
T0 = 25+T00;
r_inf = R0*exp(-B/T0);
T = B/log(R/r_inf)-T00;

== matlab function FOSWEC2/Sensor Inputs/Ohms to C1 ==
  data: R input; T output
function T = ohms2C(R)

R0 = 50000;
B = 3970;
T00 = 273.15;
T0 = 25+T00;
r_inf = R0*exp(-B/T0);
T = B/log(R/r_inf)-T00;

== matlab function FOSWEC2/FeedbackControl/MATLAB Function ==
  data: controllerType input; IctrlAft output; x input; time input; ManualGains input; Kt input; GearRatio input; GainTstep input; ExcelGains input; IctrlBow output; gainInfo output
function [IctrlAft, IctrlBow, gainInfo] = fcn(controllerType, x, time, ManualGains, Kt, GearRatio, GainTstep, ExcelGains)
% performs matrix control
% GainTstep: time step at which gains change for excel input
% Excel aft and bow matrix gain format: [Kp, Ki, CC_KP, CC_KI], time steps
% each row

IctrlAft = 0;
IctrlBow = 0;
gainInfo = zeros(4,2);
gainMat = zeros(2,4);

if controllerType == 1  % manual PI control

    B = (ManualGains * x) ./ Kt ./ GearRatio.^2;
    gainInfo = ManualGains';

elseif controllerType == 2

    idx = ceil(time./GainTstep); % Find index of current gain step
    while idx > length(ExcelGains(:,1))
        idx = idx-length(ExcelGains(:,1));
    end
    gainMat(1,1) = ExcelGains(idx,1);
    gainMat(1,2) = ExcelGains(idx,2);
    gainMat(1,3) = ExcelGains(idx,3);
    gainMat(1,4) = ExcelGains(idx,4);
    gainMat(2,1) = ExcelGains(idx,5);
    gainMat(2,2) = ExcelGains(idx,6);
    gainMat(2,3) = ExcelGains(idx,7);
    gainMat(2,4) = ExcelGains(idx,8);

    B = (gainMat * x) ./ Kt ./ GearRatio.^2;
    gainInfo = gainMat';
else
    B = [0;0];
end

IctrlAft = B(1);
IctrlBow = B(2);
